simulink model "seguim_linea_func"  (R2019b)
settings: Solver=FixedStepAuto  StartTime=0.0  StopTime=10.0  RelTol=1e-3  EnableMultiTasking=on
libraries: legoev3lib x7
settings Model: ExtModeTrigDuration=2  Creator=alumnopr18  LastModifiedBy=alumnopr18
settings SolverCC: PositivePriorityOrder=on
settings OptimizationCC: EnhancedBackFolding=on  PassReuseOutputArgsAs=Individual arguments  ZeroExternalMemoryAtStartup=off  ZeroInternalMemoryAtStartup=off  MaxStackSize=64  OptimizeBlockOrder=speed  DifferentSizesBufferReuse=on  OptimizationCustomize=off  EfficientTunableParamExpr=on
settings DebuggingCC: ParameterTunabilityLossMsg=error
settings HardwareCC: ProdBitPerPointer=32  ProdBitPerSizeT=32  ProdBitPerPtrDiffT=32  ProdLargestAtomicInteger=Long  ProdWordSize=32  ProdHWDeviceType=ARM Compatible->ARM 9
settings SFSimCC: MATLABDynamicMemAlloc=off
settings RTWCC: SystemTargetFile=ert.tlc  HardwareBoard=LEGO MINDSTORMS EV3  TLCOptions="-aInlineSetEventsForThisBaseRateFcn=TLC_FALSE -aSuppressMultiTaskScheduler=TLC_FALSE  -aRateBasedStepFcn=0"  TemplateMakefile=ert_default_tmf  GenerateReport=on  Toolchain=Sourcery G++ Lite v2009q3  IncludeHyperlinkInReport=on  LaunchReport=on  GenerateTraceInfo=on  GenerateTraceReport=on  GenerateTraceReportSl=on  GenerateTraceReportSf=on  GenerateTraceReportEml=on
settings CodeAppCC: ForceParamTrailComments=on  IgnoreCustomStorageClasses=off  OperatorAnnotations=on  SimulinkDataObjDesc=on  SFDataObjDesc=on  InsertBlockDesc=on
settings ERTTargetCC: SupportContinuousTime=on  SupportVariableSizeSignals=on

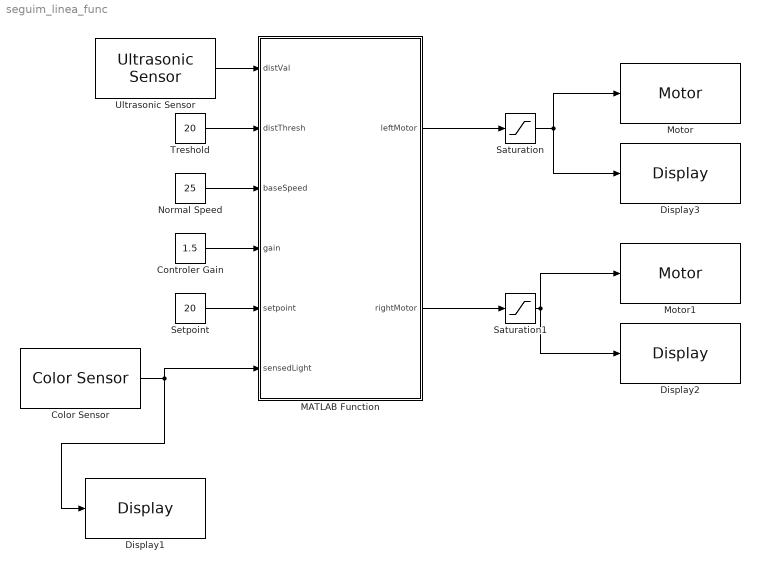
== system seguim_linea_func ==
  Color Sensor : legoev3lib/Color Sensor  portNumber=2  mode=Reflected light intensity  sampleTime=0.1
      settings: SourceProductName=Simulink Support Package for LEGO MINDSTORMS EV3 Hardware  SourceProductBaseCode=LEGOEV3
  Controler Gain : Constant  Value=1.5
  Display1 : legoev3lib/Display  slcdStr=Sensor  slcdLine=1  slcdFormat=Decimal
      settings: SourceProductName=Simulink Support Package for LEGO MINDSTORMS EV3 Hardware  SourceProductBaseCode=LEGOEV3
  Display2 : legoev3lib/Display  slcdStr=port C  slcdLine=3  slcdFormat=Decimal
      settings: SourceProductName=Simulink Support Package for LEGO MINDSTORMS EV3 Hardware  SourceProductBaseCode=LEGOEV3
  Display3 : legoev3lib/Display  slcdStr=port B  slcdLine=2  slcdFormat=Decimal
      settings: SourceProductName=Simulink Support Package for LEGO MINDSTORMS EV3 Hardware  SourceProductBaseCode=LEGOEV3
  MATLAB Function : MATLAB Function  TreatAsAtomicUnit=on
  Motor : legoev3lib/Motor  sportNumber=B  sstopAction=Brake
  Motor1 : legoev3lib/Motor  sportNumber=C  sstopAction=Brake
  Normal Speed : Constant  Value=25
  Saturation : Saturate  UpperLimit=20  LowerLimit=0
  Saturation1 : Saturate  UpperLimit=20  LowerLimit=0
  "Setpoint " : Constant  Value=20
  Treshold : Constant  Value=20
  Ultrasonic Sensor : legoev3lib/Ultrasonic Sensor  PortNumber=1  sampleTime=0.1
      settings: SourceProductName=Simulink Support Package for LEGO MINDSTORMS EV3 Hardware  SourceProductBaseCode=LEGOEV3
  wires:
  Color Sensor/1 -> Display1/1, MATLAB Function/6(sensedLight)
  Saturation/1 -> Motor/1, Display3/1
  Saturation1/1 -> Motor1/1, Display2/1
  Ultrasonic Sensor/1 -> MATLAB Function/1(distVal)
  Treshold/1 -> MATLAB Function/2(distThresh)
  Normal Speed/1 -> MATLAB Function/3(baseSpeed)
  Controler Gain/1 -> MATLAB Function/4(gain)
  "Setpoint "/1 -> MATLAB Function/5(setpoint)
  MATLAB Function/1(leftMotor) -> Saturation/1
  MATLAB Function/2(rightMotor) -> Saturation1/1

== matlab function seguim_linea_func/MATLAB Function ==
  data: distVal input; leftMotor output; distThresh input; baseSpeed input; gain input; setpoint input; sensedLight input; rightMotor output
function [leftMotor, rightMotor] = control(distVal, distThresh, baseSpeed, gain, setpoint, sensedLight)

if(distVal > distThresh) %compara la distancia del sensor al umbral
    err = sensedLight - setpoint; %lógica de seguimiento de línea
    leftMotor = err*gain;
    rightMotor = err+gain;
else
    leftMotor = uint8(0); %lógica de evitación de colisiones
    rightMotor = uint8(0);

end
